simulink model "Zcontrol_RF"  (R2016b)
settings: Solver=VariableStepAuto  StartTime=0.0  StopTime=40e-6  RelTol=1e-3
undefined symbols (not defined in the file): sigbuilder_block
libraries: simrfV2elements x11, simrfV2util1 x4, simrfV2_lib x1
settings Model: Creator=Administrator  LastModifiedBy=Administrator

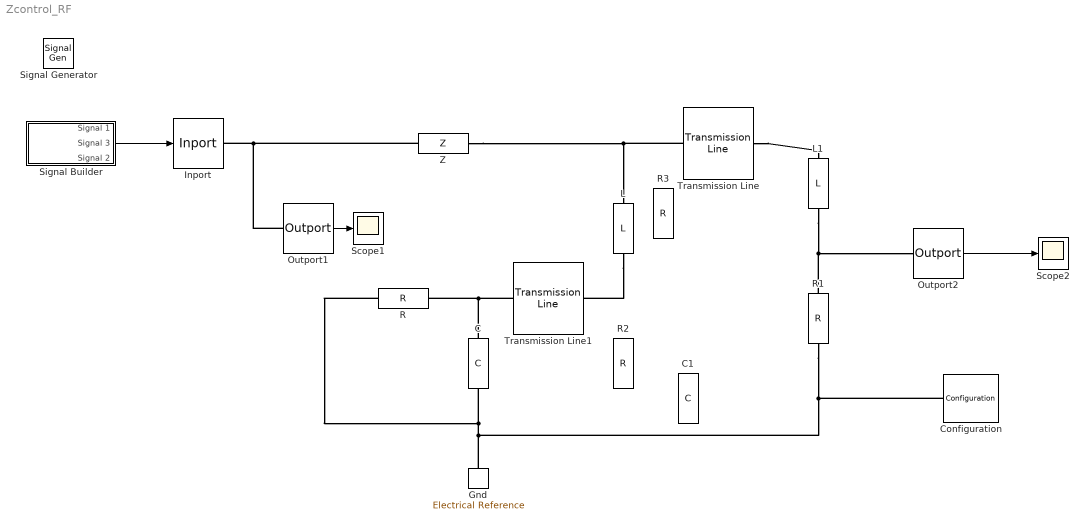
== system Zcontrol_RF ==
  C : simrfV2elements/C  classname=capacitor  Capacitance=1e-9 F
  C1 : simrfV2elements/C  classname=capacitor  Capacitance=1e-7 F
  Configuration : simrfV2util1/Configuration  AutoFreq=on  Tones=[0] Hz  Harmonics=[1]  NormalizeCarrierPower=on  SolverType=Auto  StepSize=0.01 ns  AddNoise=off  defaultRNG=on  Seed=0  Temperature=0.01 K  SolverDelFlag=0
  Gnd : simrfV2_lib/Elements/Electrical Reference
  Inport : simrfV2util1/Inport  SimulinkInputSignalType=Ideal voltage  CarrierFreq=0 Hz  ZS=0  InternalGrounding=on
  L : simrfV2elements/L  classname=inductor  Inductance=1e-3 H
  L1 : simrfV2elements/L  classname=inductor  Inductance=1e-8 H
  Outport1 : simrfV2util1/Outport  SensorType=Ideal voltage  OutputFormat=Complex Baseband  CarrierFreq=0 Hz  ZL=Inf  InternalGrounding=on  StepSize=1e-6 s  AutoStep=on
  Outport2 : simrfV2util1/Outport  SensorType=Ideal voltage  OutputFormat=Complex Baseband  CarrierFreq=0 Hz  ZL=Inf  InternalGrounding=on  StepSize=1e-6 s  AutoStep=on
  R : simrfV2elements/R  classname=resistor  Resistance=1000 Ohm  AddNoise=on
  R1 : simrfV2elements/R  classname=resistor  Resistance=0.1 Ohm  AddNoise=on
  R2 : simrfV2elements/R  classname=resistor  Resistance=50 Ohm  AddNoise=on
  R3 : simrfV2elements/R  classname=resistor  Resistance=240 Ohm  AddNoise=on
  Scope1 : Scope
  Scope2 : Scope
  Signal Generator : SignalGenerator  WaveForm=square  Frequency=0.2e5
  Signal Builder : Subsystem  Tag=STV Subsys  LoadFcn=sigbuilder_block('load');  StartFcn=sigbuilder_block('start');  StopFcn=sigbuilder_block('stop');  ClipboardFcn=sigbuilder_block('clipboard');  mask(Sigbuilder block){tuvar=[0:10]}
      mask help: Simulink:masks:SigbuilderBlock_MD
      mask init:
      | if ~strcmp(get_param(bdroot(gcbh),'SimulationStatus'),'stopped') tuvar = sigbuilder_block('maskInit'); end
      settings: CopyFcn=sigbuilder_block('copy');  DeleteFcn=sigbuilder_block('delete');  ModelCloseFcn=sigbuilder_block('modelClose');  PreSaveFcn=sigbuilder_block('preSave');  PauseFcn=sigbuilder_block('pause');  ContinueFcn=sigbuilder_block('continue');  NameChangeFcn=sigbuilder_block('namechange');  OpenFcn=sigbuilder_block('open',[0 28.8 1152 564.6 ]);  CloseFcn=sigbuilder_block('close');
      mask Display: plot(0, 0, 100, 100,[2, 2, 32, 32, 2], [68, 8, 8, 68, 68],[32, 2], [38, 38], [32, 19, 2],[53, 60, 44], [32, 17, 17, 2],[16, 16, 31, 31]);txt = getActiveGroup(gcbh);text(2, 100, txt,'verticalAlignment', 'top');
  Transmission Line : simrfV2elements/Transmission Line  classname=xline  Model_type=Delay-based and lossless  Parameterization=By characteristic impedance and capacitance  TransDelay=1.3e-9 s  CharImped=50 Ohm  Resistance=.3 Ohm/m  Inductance=235e-9 H/m  Capacitance=94e-12 F/m  Conductance=5e-6 S/m  LineLength=1 cm  NumSegments=10  InternalGrounding=on  OuterRadius=2.57 mm  InnerRadius=0.725 mm  MuR=1  EpsilonR=2.2  LossTangent=0  SigmaCond=inf S/m  StubMode=Not a stub  Termination=Open  ConductorWidth=0.6 mm  SlotWidth=0.2 mm  Height=0.635 mm  Thickness=5 um  SWidth=0.6 mm  Radius=0.67 mm  Separation=1.62 mm  PWidth=5 mm  PSeparation=1 mm  PV=299792458  Loss=0  SourceFreq=User-specified  PlotFreq=[1e9:1e6:3e9] Hz  PlotType=X-Y plane  YParam1=S11  YFormat1=Magnitude (decibels)  YParam2=S22  YFormat2=Magnitude (decibels)  YOption=Linear  XOption=Linear  FitOpt=Share all poles  FitTol=-40  SparamRepresentation=Frequency domain  Freq=1e9 Hz  Interp_type=Linear  AutoImpulseLength=off  ImpulseLength=0 s
  Transmission Line1 : simrfV2elements/Transmission Line  classname=xline  Model_type=Delay-based and lossless  Parameterization=By characteristic impedance and capacitance  TransDelay=5e-9 s  CharImped=50 Ohm  Resistance=.3 Ohm/m  Inductance=235e-9 H/m  Capacitance=94e-12 F/m  Conductance=5e-6 S/m  LineLength=1 cm  NumSegments=10  InternalGrounding=on  OuterRadius=2.57 mm  InnerRadius=0.725 mm  MuR=1  EpsilonR=2.2  LossTangent=0  SigmaCond=inf S/m  StubMode=Not a stub  Termination=Open  ConductorWidth=0.6 mm  SlotWidth=0.2 mm  Height=0.635 mm  Thickness=5 um  SWidth=0.6 mm  Radius=0.67 mm  Separation=1.62 mm  PWidth=5 mm  PSeparation=1 mm  PV=299792458  Loss=0  SourceFreq=User-specified  PlotFreq=[1e9:1e6:3e9] Hz  PlotType=X-Y plane  YParam1=S11  YFormat1=Magnitude (decibels)  YParam2=S22  YFormat2=Magnitude (decibels)  YOption=Linear  XOption=Linear  FitOpt=Share all poles  FitTol=-40  SparamRepresentation=Frequency domain  Freq=1e9 Hz  Interp_type=Linear  AutoImpulseLength=off  ImpulseLength=0 s
  Z : simrfV2elements/Z  classname=complex_impedance  Impedance_type=Frequency independent  Impedance=50  Freq=1e9 Hz
  wires:
  Outport1/1 -> Scope1/1
  Outport2/1 -> Scope2/1
  Signal Builder/2(Signal 3) -> Inport/1
  connections:
  C/LConn1 -- R/RConn1 -- Transmission Line1/LConn1
  Configuration/LConn1 -- R/LConn1 -- C/RConn1 -- Gnd/LConn1 -- R1/RConn1
  Z/LConn1 -- Outport1/LConn1 -- Inport/RConn1
  Z/RConn1 -- Transmission Line/LConn1 -- L/LConn1
  R1/LConn1 -- L1/RConn1 -- Outport2/LConn1
  L/RConn1 -- Transmission Line1/RConn1
  Transmission Line/RConn1 -- L1/LConn1

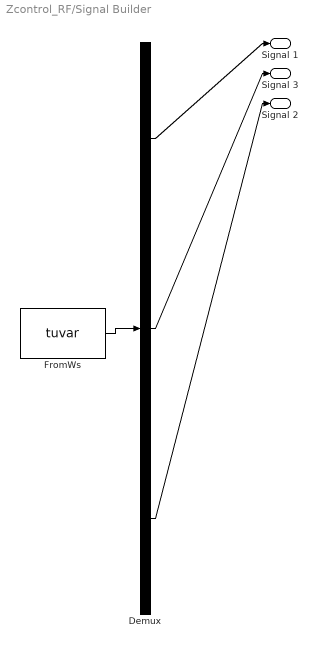
== system Zcontrol_RF/Signal Builder ==
  Demux : Demux  Tag=STV Demux  Outputs=3
  FromWs : FromWorkspace  Tag=STV FromWs  VariableName=tuvar  SampleTime=0
      SigBuilderData=|
      | common.afterFinalStr = 'Extrapolate'
      | common.sampleTime = 0
      | dataSet.timeRange = [0 4e-05]
      | dataSet.name = 'Group 1'
      | sbobj.Groups.Name = 'Group 1'
      | sbobj.Groups.Signals(1).Name = 'Signal 1'
      | sbobj.Groups.Signals(1).XData = [0 4e-07 4.02e-07 5e-07 5.02e-07 4e-05]
      | sbobj.Groups.Signals(1).YData = [1 0 1 1 0 0]
      | sbobj.Groups.Signals(2).Name = 'Signal 3'
      | sbobj.Groups.Signals(2).XData = [0 2e-05 2.0002e-05 4e-05]
      | sbobj.Groups.Signals(2).YData = [1 1 0 0]
      | sbobj.Groups.Signals(3).Name = 'Signal 2'
      | sbobj.Groups.Signals(3).XData = [0 1e-05 4e-05]
      | sbobj.Groups.Signals(3).YData = [1 1 0.999]
      | sbobj.Groups.TimeRange = [0 4e-05]
  Signal 1 : Outport  Tag=STV Outport
  Signal 3 : Outport  Tag=STV Outport  Port=2
  Signal 2 : Outport  Tag=STV Outport  Port=3
  wires:
  FromWs/1 -> Demux/1
  Demux/1 -> Signal 1/1
  Demux/2 -> Signal 3/1
  Demux/3 -> Signal 2/1
